simulink model "repo2_5"  (R2019a)
settings: Solver=VariableStepAuto  StartTime=0.0  StopTime=40.0  RelTol=1e-3
settings Model: Creator=toshi  LastModifiedBy=toshi

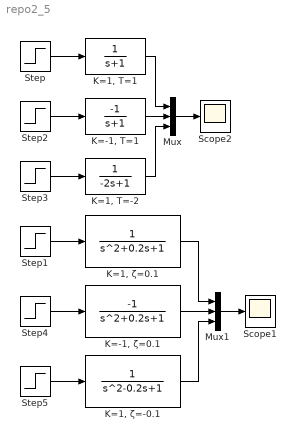
== system repo2_5 ==
  "K=-1, T=1" : TransferFcn  Numerator=[-1]  Denominator=[1 1]
  "K=-1, ζ=0.1" : TransferFcn  Numerator=[-1]  Denominator=[1 0.2 1]
  "K=1, T=-2" : TransferFcn  Denominator=[-2 1]
  "K=1, T=1" : TransferFcn  Denominator=[1 1]
  "K=1, ζ=-0.1" : TransferFcn  Denominator=[1 -0.2 1]
  "K=1, ζ=0.1" : TransferFcn  Denominator=[1 0.2 1]
  Mux : Mux  Inputs=3
  Mux1 : Mux  Inputs=3
  Scope1 : Scope
  Scope2 : Scope
  Step{,1..5} (6 alike) : Step  SampleTime=0
  wires:
  "K=1, T=1"/1 -> Mux/1
  Step/1 -> "K=1, T=1"/1
  Step1/1 -> "K=1, ζ=0.1"/1
  Step2/1 -> "K=-1, T=1"/1
  "K=-1, T=1"/1 -> Mux/2
  Mux/1 -> Scope2/1
  Step3/1 -> "K=1, T=-2"/1
  "K=1, T=-2"/1 -> Mux/3
  Step4/1 -> "K=-1, ζ=0.1"/1
  Step5/1 -> "K=1, ζ=-0.1"/1
  "K=1, ζ=0.1"/1 -> Mux1/1
  Mux1/1 -> Scope1/1
  "K=-1, ζ=0.1"/1 -> Mux1/2
  "K=1, ζ=-0.1"/1 -> Mux1/3
